simulink library "laser_library"  (Simulink 7.5)
settings: Solver=ode45  StartTime=0.0  StopTime=10.0  RelTol=1e-3
libraries: simulink x3, aerolibutil x3, falter_library x2, aerolibtransform2 x1
settings Model: Creator=elm  LastModifiedBy=falter

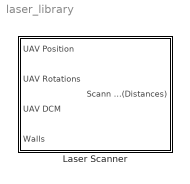
== system laser_library ==
  Laser Scanner : Subsystem  mask{scannerParameters=[0 0 0 1 0 0]}
      mask prompts: scannerParameters "Scanner Parameters"

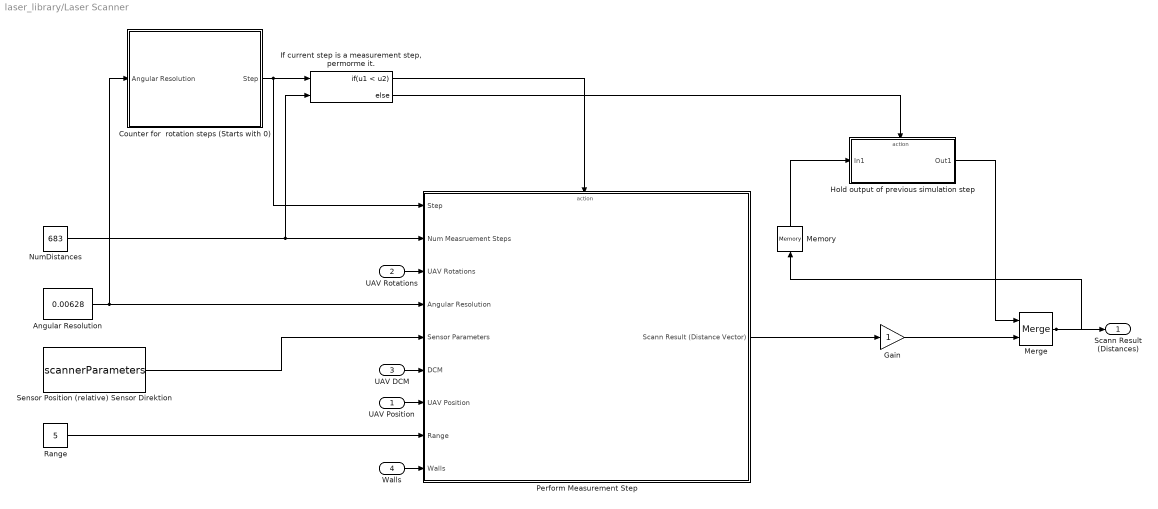
== system laser_library/Laser Scanner ==
  UAV Position : Inport  SampleTime=0.0001
  UAV Rotations : Inport  Port=2  SampleTime=0.0001
  UAV DCM : Inport  Port=3  SampleTime=0.0001
  Walls : Inport  Port=4  SampleTime=0.0001
  Angular Resolution : Constant  Value=0.00628  OutDataType=fixdt(1, 16)  OutScaling=2^0
  Counter for  rotation steps (Starts with 0) : Subsystem
  Gain : Gain  ParameterDataType=fixdt(1, 16)  ParameterScaling=2^0  OutDataType=fixdt(1, 16)  OutScaling=2^0
  Hold output of previous simulation step : Subsystem  TreatAsAtomicUnit=on
  "If current step is a measurement step, permorme it." : If  NumInputs=2  IfExpression=u1 < u2
  Memory : Memory
  Merge : Merge  InitialOutput=0
  NumDistances : Constant  Value=683  OutDataType=fixdt(1, 16)  OutScaling=2^0
  Perform Measurement Step : Subsystem
  Range : Constant  Value=5  OutDataType=fixdt(1, 16)  OutScaling=2^0
  Sensor Position (relative) Sensor Direktion : Constant  Value=scannerParameters  OutDataType=fixdt(1, 16)  OutScaling=2^0
  Scann Result (Distances) : Outport  SampleTime=0.0001
  wires:
  Sensor Position (relative) Sensor Direktion/1 -> Perform Measurement Step/5(Sensor Parameters)
  Walls/1 -> Perform Measurement Step/9(Walls)
  UAV Position/1 -> Perform Measurement Step/7(UAV Position)
  UAV DCM/1 -> Perform Measurement Step/6(DCM)
  UAV Rotations/1 -> Perform Measurement Step/3(UAV Rotations)
  Gain/1 -> Merge/2
  Memory/1 -> Hold output of previous simulation step/1(In1)
  Merge/1 -> Scann Result (Distances)/1, Memory/1
  Hold output of previous simulation step/1(Out1) -> Merge/1
  "If current step is a measurement step, permorme it."/2 -> Hold output of previous simulation step/Action
  Perform Measurement Step/1(Scann Result (Distance Vector)) -> Gain/1
  "If current step is a measurement step, permorme it."/1 -> Perform Measurement Step/Action
  Counter for  rotation steps (Starts with 0)/1(Step) -> Perform Measurement Step/1(Step), "If current step is a measurement step, permorme it."/1
  NumDistances/1 -> Perform Measurement Step/2(Num Measruement Steps), "If current step is a measurement step, permorme it."/2
  Range/1 -> Perform Measurement Step/8(Range)
  Angular Resolution/1 -> Counter for  rotation steps (Starts with 0)/1(Angular Resolution), Perform Measurement Step/4(Angular Resolution)

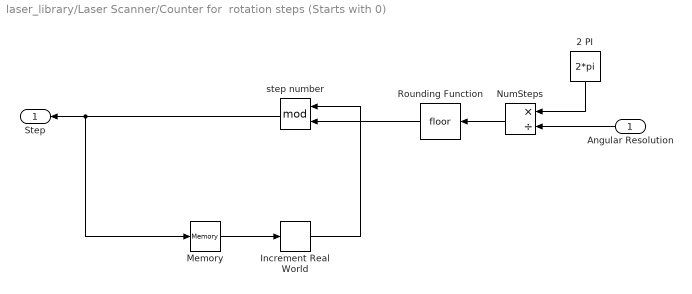
== system laser_library/Laser Scanner/Counter for  rotation steps (Starts with 0) ==
  Angular Resolution : Inport  OutDataType=fixdt(1, 16)  OutScaling=2^0
  2 PI : Constant  Value=2*pi  OutDataType=fixdt(1, 16)  OutScaling=2^0
  Increment Real World : simulink/Additional Math & Discrete/Additional Math: Increment - Decrement/Increment Real World  SystemSampleTime=-1
  Memory : Memory  InheritSampleTime=on
  NumSteps : Product  Inputs=*/  OutDataType=fixdt(1, 16)  OutScaling=2^-10
  Rounding Function : Rounding
  step number : Math  Operator=mod  OutDataType=fixdt(1, 16)  OutScaling=2^0  SaturateOnIntegerOverflow=on
  Step : Outport
  wires:
  Rounding Function/1 -> step number/2
  NumSteps/1 -> Rounding Function/1
  2 PI/1 -> NumSteps/1
  Angular Resolution/1 -> NumSteps/2
  step number/1 -> Memory/1, Step/1
  Increment Real World/1 -> step number/1
  Memory/1 -> Increment Real World/1

== system laser_library/Laser Scanner/Hold output of previous simulation step ==
  In1 : Inport  OutDataType=fixdt(1, 16)  OutScaling=2^0
  Action Port : ActionPort
  Out1 : Outport  OutDataType=fixdt(1, 16)  OutScaling=2^0  InitialOutput=0
  wires:
  In1/1 -> Out1/1

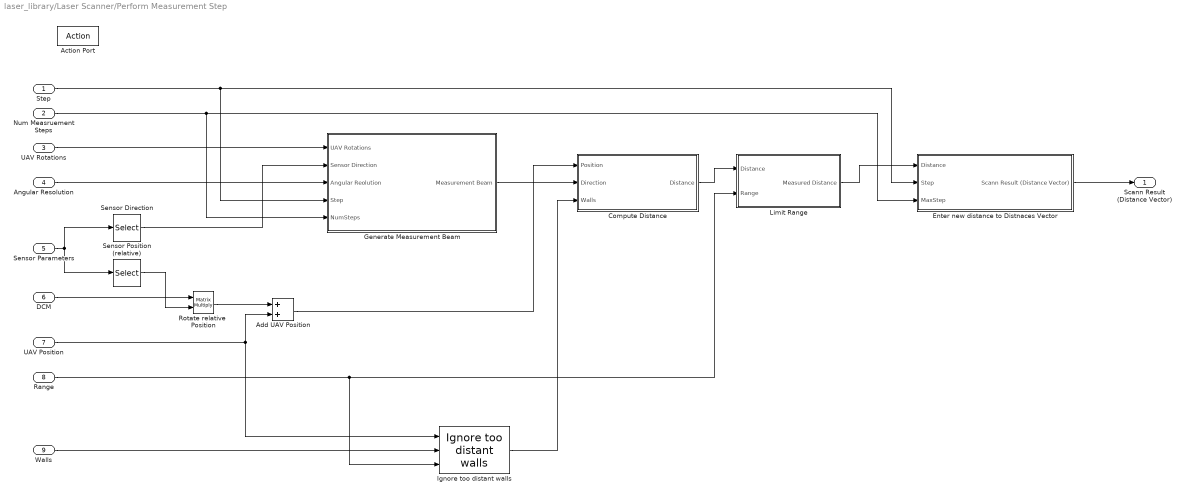
== system laser_library/Laser Scanner/Perform Measurement Step ==
  Step : Inport
  Num Measruement Steps : Inport  Port=2
  UAV Rotations : Inport  Port=3
  Angular Resolution : Inport  Port=4
  Sensor Parameters : Inport  Port=5
  DCM : Inport  Port=6
  UAV Position : Inport  Port=7
  Range : Inport  Port=8
  Walls : Inport  Port=9
  Action Port : ActionPort
  Add UAV Position : Sum  OutDataType=fixdt(1, 16)  OutScaling=2^-10
  Compute Distance : Subsystem
  Enter new distance to Distnaces Vector : Subsystem
  Generate Measurement Beam : Subsystem
  Ignore too distant walls : falter_library/Ignore too distant walls  SystemSampleTime=-1
  Limit Range : Subsystem
  Rotate relative  Position : Product  Multiplication=Matrix(*)  OutDataType=fixdt(1, 16)  OutScaling=2^0  RndMeth=Zero
  Sensor Direction : Selector  InputPortWidth=6  IndexOptions=Index vector (dialog)  Indices=[4 5 6]  OutputSizes=1
  Sensor Position (relative) : Selector  InputPortWidth=6  IndexOptions=Index vector (dialog)  Indices=[1 2 3]  OutputSizes=1
  Scann Result (Distance Vector) : Outport  InitialOutput=0
  wires:
  Walls/1 -> Ignore too distant walls/2
  Ignore too distant walls/1 -> Compute Distance/3(Walls)
  Angular Resolution/1 -> Generate Measurement Beam/3(Angular Reolution)
  Enter new distance to Distnaces Vector/1(Scann Result (Distance Vector)) -> Scann Result (Distance Vector)/1
  UAV Rotations/1 -> Generate Measurement Beam/1(UAV Rotations)
  Num Measruement Steps/1 -> Generate Measurement Beam/5(NumSteps), Enter new distance to Distnaces Vector/3(MaxStep)
  Limit Range/1(Measured Distance) -> Enter new distance to Distnaces Vector/1(Distance)
  Compute Distance/1(Distance) -> Limit Range/1(Distance)
  Range/1 -> Limit Range/2(Range), Ignore too distant walls/3
  Step/1 -> Enter new distance to Distnaces Vector/2(Step), Generate Measurement Beam/4(Step)
  Generate Measurement Beam/1(Measurement Beam) -> Compute Distance/2(Direction)
  Add UAV Position/1 -> Compute Distance/1(Position)
  UAV Position/1 -> Add UAV Position/2, Ignore too distant walls/1
  Sensor Direction/1 -> Generate Measurement Beam/2(Sensor Direction)
  Sensor Parameters/1 -> Sensor Direction/1, Sensor Position (relative)/1
  DCM/1 -> Rotate relative  Position/1
  Sensor Position (relative)/1 -> Rotate relative  Position/2
  Rotate relative  Position/1 -> Add UAV Position/1

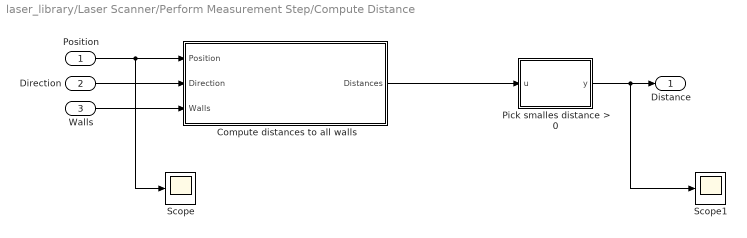
== system laser_library/Laser Scanner/Perform Measurement Step/Compute Distance ==
  Position : Inport  OutDataType=fixdt(1, 16)  OutScaling=2^0
  Direction : Inport  Port=2  OutDataType=fixdt(1, 16)  OutScaling=2^0
  Walls : Inport  Port=3  OutDataType=fixdt(1, 16)  OutScaling=2^0
  Compute distances to all walls : Subsystem  TreatAsAtomicUnit=on
  Pick smalles distance > 0 : Stateflow chart  TreatAsAtomicUnit=on
  Scope : Scope
      settings: YMin=0  YMax=1  SaveName=ScopeData4
  Scope1 : Scope
      settings: YMin=0  YMax=130  SaveName=ScopeData3
  Distance : Outport  OutDataType=fixdt(1, 16)  OutScaling=2^0
  wires:
  Pick smalles distance > 0/1(y) -> Distance/1, Scope1/1
  Compute distances to all walls/1(Distances) -> Pick smalles distance > 0/1(u)
  Position/1 -> Scope/1, Compute distances to all walls/1(Position)
  Direction/1 -> Compute distances to all walls/2(Direction)
  Walls/1 -> Compute distances to all walls/3(Walls)

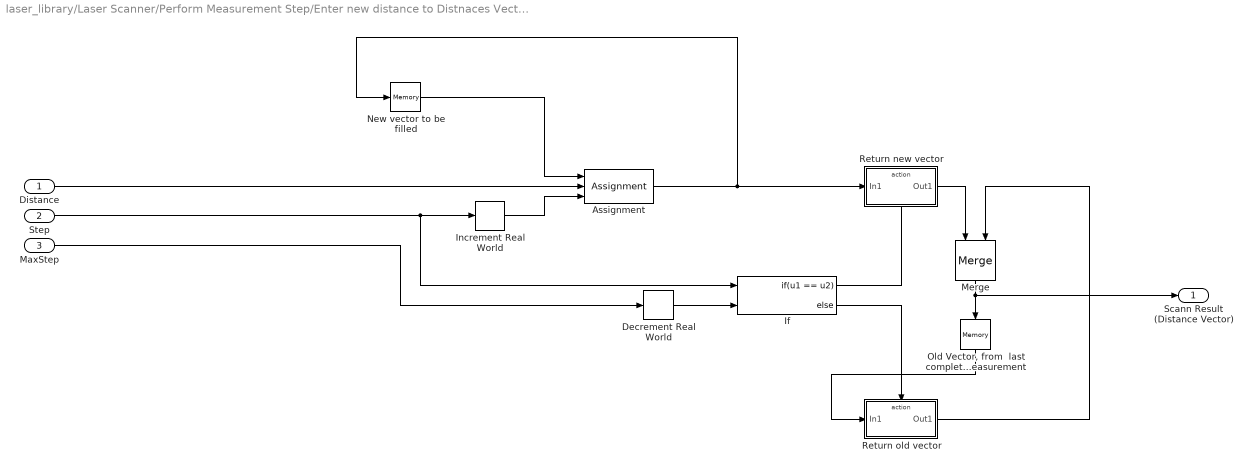
== system laser_library/Laser Scanner/Perform Measurement Step/Enter new distance to Distnaces Vector ==
  Distance : Inport  OutDataType=fixdt(1, 16)  OutScaling=2^0
  Step : Inport  Port=2  OutDataType=fixdt(1, 16)  OutScaling=2^0
  MaxStep : Inport  Port=3  OutDataType=fixdt(1, 16)  OutScaling=2^0
  Assignment : Assignment  IndexOptions=Index vector (port)  Indices=1  OutputSizes=1
  Decrement Real World : simulink/Additional Math & Discrete/Additional Math: Increment - Decrement/Decrement Real World  SystemSampleTime=-1
  If : If  NumInputs=2  IfExpression=u1 == u2
  Increment Real World : simulink/Additional Math & Discrete/Additional Math: Increment - Decrement/Increment Real World  SystemSampleTime=-1
  Merge : Merge  InitialOutput=0
  New vector to be filled : Memory  X0=[0 0 0 0 0 0 0 0 0 0 0 0 0 0 0 0 0 0 0 0 0 0 0 0 0 0 0 0 0 0 0 0 0 0 0 0 0 0 0 0 0 0 0 0 0 0 0 0 0 0 0 0 0 0 0 0 0 0 0 0 0 0 0 0 0 0 0 0 0 0 0 0 0 0 0 0 0 0 0 0 0 0 0 0 0 0 0 0 0 0 0 0 0 0 0 0 0 0 0 0 0 0 0 0 0 0 0 0 0 0 0 0 0 0 0 0 0 0 0 0 0 0 0 0 0 0 0 0 0 0 0 0 0 0 0 0 0 0 0 0 0 0 0 0 0 0 0 0 0 0 0 0 0 0 0 0 0 0 0 0 0 0 0 0 0 0 0 0 0 0 0 0 0 0 0 0 0 0 0 0 0 0 0 0 0 0 0 0 0 0 0 0 0 0 0 0 0 0 0 0 0 0 0 0 0 0 0 0 0 0 0 0 0 0 0 0 0 0 0 0 0 0 0 0 0 0 0 0 0 0 0 0 0 0 0 0 0 0 0 0 0 0 0 0 0 0 0 0 0 0 0 0 0 0 0 0 0 0 0 0 0 0 0 0 0 0 0 0 0 0 0 0 0 0 0 0 0 0 0 0 0 0 0 0 0 0 0 0 0 0 0 0 0 0 0 0 0 0 0 0 0 0 0 0 0 0 0 0 0 0 0 0 0 0 0 0 0 0 0 0 0 0 0 0 0 0 0 0 0 0 0 0 0 0 0 0 0 0 0 0 0 0 0 0 0 0 0 0 0 0 0 0 0 0 0 0 0 0 0 0 0 0 0 0 0 0 0 0 0 0 0 0 0 0 0 0 0 0 0 0 0 0 0 0 0 0 0 0 0 0 0 0 0 0 0 0 0 0 0 0 0 0 0 0 0 0 0 0 0 0 0 0 0 0 0 0 0 0 0 0 0 0 0 0 0 0 0 0 0 0 0 0 0 0 0 0 0 0 0 0 0 0 0 0 0 0 0 0 0 0 0 0 0 0 0 0 0 0 0 0 0 0 0 0 0 0 0 0 0 0 0 0 0 0 0 0 0 0 0 0 0 0 0 0 0 0 0 0 0 0 0 0 0 0 0 0 0 0 0 0 0 0 0 0 0 0 0 0 0 0 0 0 0 0 0 0 0 0 0 0 0 0 0 0 0 0 0 0 0 0 0 0 0 0 0 0 0 0 0 0 0 0 0 0 0 0 0 0 0 0 0 0 0 0 0 0 0 0 0 0 0 0 0 0 0 0 0 0 0 0 0 0 0 0 0 0 0 0 0 0 0 0 0 0 0 0 0 0 0 0 0 0 0 0 0 0 0 0 0 0 0 0 0 0 0 0 0 0 0 0 0 0 0 0 0 0 0 0 0 0 0 0 0 0 0 0 0 0 0 0 0 0 0 0 0 0 0 0 0 0 0 0 0 0 0 0 0 0 0 0 0 0 0 0 0 0 0 0 0 0 0 0 0 0 0 0 0 0 0 0 0 0 0 0 0 0 0 0 0 0 0 0 0]  InheritSampleTime=on
  "Old Vector, from  last complete  measurement" : Memory  X0=[0 0 0 0 0 0 0 0 0 0 0 0 0 0 0 0 0 0 0 0 0 0 0 0 0 0 0 0 0 0 0 0 0 0 0 0 0 0 0 0 0 0 0 0 0 0 0 0 0 0 0 0 0 0 0 0 0 0 0 0 0 0 0 0 0 0 0 0 0 0 0 0 0 0 0 0 0 0 0 0 0 0 0 0 0 0 0 0 0 0 0 0 0 0 0 0 0 0 0 0 0 0 0 0 0 0 0 0 0 0 0 0 0 0 0 0 0 0 0 0 0 0 0 0 0 0 0 0 0 0 0 0 0 0 0 0 0 0 0 0 0 0 0 0 0 0 0 0 0 0 0 0 0 0 0 0 0 0 0 0 0 0 0 0 0 0 0 0 0 0 0 0 0 0 0 0 0 0 0 0 0 0 0 0 0 0 0 0 0 0 0 0 0 0 0 0 0 0 0 0 0 0 0 0 0 0 0 0 0 0 0 0 0 0 0 0 0 0 0 0 0 0 0 0 0 0 0 0 0 0 0 0 0 0 0 0 0 0 0 0 0 0 0 0 0 0 0 0 0 0 0 0 0 0 0 0 0 0 0 0 0 0 0 0 0 0 0 0 0 0 0 0 0 0 0 0 0 0 0 0 0 0 0 0 0 0 0 0 0 0 0 0 0 0 0 0 0 0 0 0 0 0 0 0 0 0 0 0 0 0 0 0 0 0 0 0 0 0 0 0 0 0 0 0 0 0 0 0 0 0 0 0 0 0 0 0 0 0 0 0 0 0 0 0 0 0 0 0 0 0 0 0 0 0 0 0 0 0 0 0 0 0 0 0 0 0 0 0 0 0 0 0 0 0 0 0 0 0 0 0 0 0 0 0 0 0 0 0 0 0 0 0 0 0 0 0 0 0 0 0 0 0 0 0 0 0 0 0 0 0 0 0 0 0 0 0 0 0 0 0 0 0 0 0 0 0 0 0 0 0 0 0 0 0 0 0 0 0 0 0 0 0 0 0 0 0 0 0 0 0 0 0 0 0 0 0 0 0 0 0 0 0 0 0 0 0 0 0 0 0 0 0 0 0 0 0 0 0 0 0 0 0 0 0 0 0 0 0 0 0 0 0 0 0 0 0 0 0 0 0 0 0 0 0 0 0 0 0 0 0 0 0 0 0 0 0 0 0 0 0 0 0 0 0 0 0 0 0 0 0 0 0 0 0 0 0 0 0 0 0 0 0 0 0 0 0 0 0 0 0 0 0 0 0 0 0 0 0 0 0 0 0 0 0 0 0 0 0 0 0 0 0 0 0 0 0 0 0 0 0 0 0 0 0 0 0 0 0 0 0 0 0 0 0 0 0 0 0 0 0 0 0 0 0 0 0 0 0 0 0 0 0 0 0 0 0 0 0 0 0 0 0 0 0 0 0 0 0 0 0 0 0 0 0 0 0 0 0 0 0 0 0 0 0 0 0 0 0 0 0 0 0 0 0 0 0 0 0 0 0 0 0 0 0 0 0 0 0 0 0 0 0 0 0 0 0 0 0 0 0 0 0 0]  InheritSampleTime=on
  Return new vector : Subsystem  TreatAsAtomicUnit=on
  Return old vector : Subsystem  TreatAsAtomicUnit=on
  Scann Result (Distance Vector) : Outport  OutDataType=fixdt(1, 16)  OutScaling=2^0
  wires:
  Decrement Real World/1 -> If/2
  Return old vector/1(Out1) -> Merge/2
  Merge/1 -> Scann Result (Distance Vector)/1, "Old Vector, from  last complete  measurement"/1
  Return new vector/1(Out1) -> Merge/1
  Distance/1 -> Assignment/2
  "Old Vector, from  last complete  measurement"/1 -> Return old vector/1(In1)
  If/2 -> Return old vector/Action
  If/1 -> Return new vector/Action
  MaxStep/1 -> Decrement Real World/1
  Assignment/1 -> New vector to be filled/1, Return new vector/1(In1)
  Step/1 -> If/1, Increment Real World/1
  New vector to be filled/1 -> Assignment/1
  Increment Real World/1 -> Assignment/3

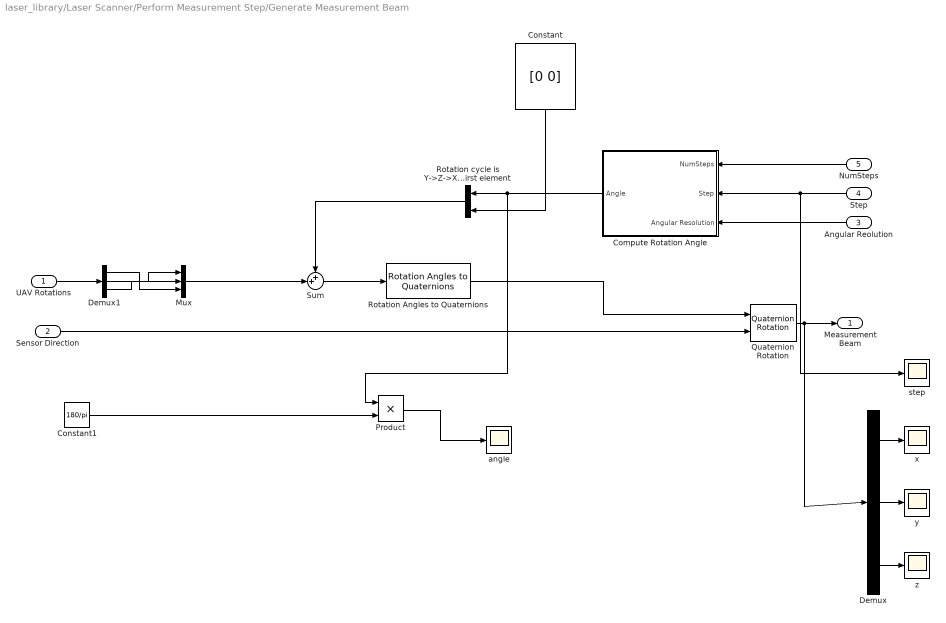
== system laser_library/Laser Scanner/Perform Measurement Step/Generate Measurement Beam ==
  UAV Rotations : Inport
  Sensor Direction : Inport  Port=2
  Angular Reolution : Inport  Port=3
  Step : Inport  Port=4
  NumSteps : Inport  Port=5
  Compute Rotation Angle : Subsystem
  Constant : Constant  Value=[0 0]  OutDataType=fixdt(1, 16)  OutScaling=2^0
  Constant1 : Constant  Value=180/pi  OutDataType=fixdt(1, 16)  OutScaling=2^0
  Demux : Demux  Outputs=3
  Demux1 : Demux  Outputs=3
  Mux : Mux  Inputs=3
  Product : Product  OutDataType=fixdt(1, 16)  OutScaling=2^0  RndMeth=Zero
  Quaternion Rotation : aerolibutil/Quaternion Rotation  SystemSampleTime=-1
  Rotation Angles to Quaternions : aerolibtransform2/Rotation Angles to Quaternions  SystemSampleTime=-1  rotationOrder=YZX
  Rotation cycle is Y->Z->X y (vertical ax. in sim!) is first element : Concatenate  Mode=Vector
  Sum : Sum  Inputs=++|  OutDataType=fixdt(1, 16)  OutScaling=2^0
  angle : Scope
      settings: YMin=0  YMax=700  SaveName=ScopeData5
  step : Scope
      settings: YMin=0  YMax=700
  x : Scope
      settings: YMin=-2.5  YMax=2.5  SaveName=ScopeData2
  y : Scope
      settings: YMin=-1  YMax=1  SaveName=ScopeData4
  z : Scope
      settings: YMin=-1  YMax=1  SaveName=ScopeData3
  Measurement Beam : Outport
  wires:
  NumSteps/1 -> Compute Rotation Angle/1(NumSteps)
  Step/1 -> Compute Rotation Angle/2(Step), step/1
  Angular Reolution/1 -> Compute Rotation Angle/3(Angular Resolution)
  Sensor Direction/1 -> Quaternion Rotation/2
  Sum/1 -> Rotation Angles to Quaternions/1
  Rotation Angles to Quaternions/1 -> Quaternion Rotation/1
  Rotation cycle is Y->Z->X y (vertical ax. in sim!) is first element/1 -> Sum/1
  Demux/1 -> x/1
  Demux/2 -> y/1
  Demux/3 -> z/1
  Quaternion Rotation/1 -> Measurement Beam/1, Demux/1
  Compute Rotation Angle/1(Angle) -> Rotation cycle is Y->Z->X y (vertical ax. in sim!) is first element/1, Product/1
  Constant/1 -> Rotation cycle is Y->Z->X y (vertical ax. in sim!) is first element/2
  Constant1/1 -> Product/2
  Product/1 -> angle/1
  UAV Rotations/1 -> Demux1/1
  Demux1/1 -> Mux/3
  Demux1/2 -> Mux/1
  Demux1/3 -> Mux/2
  Mux/1 -> Sum/2

== system laser_library/Laser Scanner/Perform Measurement Step/Limit Range ==
  Distance : Inport  OutDataType=fixdt(1, 16)  OutScaling=2^0
  Range : Inport  Port=2  OutDataType=fixdt(1, 16)  OutScaling=2^0
  If : If  NumInputs=2  IfExpression=u1 <= u2
  If Action Subsystem : Subsystem  TreatAsAtomicUnit=on
  If Action Subsystem1 : Subsystem  TreatAsAtomicUnit=on
  Merge : Merge  InitialOutput=0
  Measured Distance : Outport  OutDataType=fixdt(1, 16)  OutScaling=2^0
  wires:
  Merge/1 -> Measured Distance/1
  If Action Subsystem1/1(Distance=0) -> Merge/2
  If Action Subsystem/1(Out) -> Merge/1
  If/2 -> If Action Subsystem1/Action
  If/1 -> If Action Subsystem/Action
  Range/1 -> If/2
  Distance/1 -> If Action Subsystem/1(In), If/1

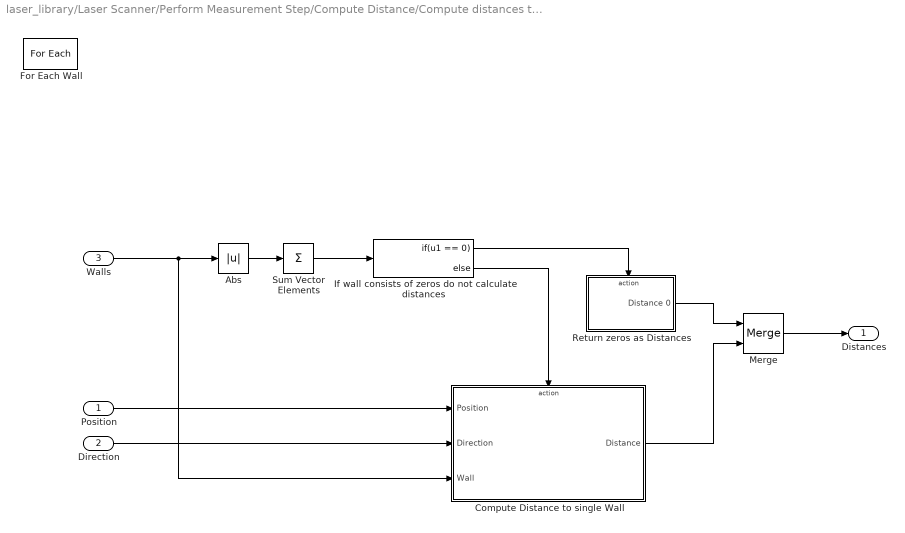
== system laser_library/Laser Scanner/Perform Measurement Step/Compute Distance/Compute distances to all walls ==
  Position : Inport  OutDataType=fixdt(1, 16)  OutScaling=2^0  Partition=off
  Direction : Inport  Port=2  OutDataType=fixdt(1, 16)  OutScaling=2^0  Partition=off
  Walls : Inport  Port=3  OutDataType=fixdt(1, 16)  OutScaling=2^0  Partition=on  PartitionDimension=1  PartitionWidth=1
  Abs : Abs  OutDataType=fixdt(1, 16)  OutScaling=2^0
  Compute Distance to single Wall : Subsystem
  For Each Wall : ForEach  DisableCoverage=on  IndexMode=One-based
  If wall consists of zeros do not calculate distances : If  IfExpression=u1 == 0
  Merge : Merge  InitialOutput=0
  Return zeros as Distances : Subsystem  TreatAsAtomicUnit=on
  Sum Vector Elements : Sum  Inputs=+  OutDataType=fixdt(1, 16)  OutScaling=2^-10
  Distances : Outport  OutDataType=fixdt(1, 16)  OutScaling=2^0  ConcatenationDimension=1
  wires:
  If wall consists of zeros do not calculate distances/2 -> Compute Distance to single Wall/Action
  Compute Distance to single Wall/1(Distance) -> Merge/2
  Sum Vector Elements/1 -> If wall consists of zeros do not calculate distances/1
  Merge/1 -> Distances/1
  Return zeros as Distances/1(Distance 0) -> Merge/1
  Position/1 -> Compute Distance to single Wall/1(Position)
  Direction/1 -> Compute Distance to single Wall/2(Direction)
  Walls/1 -> Compute Distance to single Wall/3(Wall), Abs/1
  If wall consists of zeros do not calculate distances/1 -> Return zeros as Distances/Action
  Abs/1 -> Sum Vector Elements/1

== system laser_library/Laser Scanner/Perform Measurement Step/Enter new distance to Distnaces Vector/Return new vector ==
  In1 : Inport  OutDataType=fixdt(1, 16)  OutScaling=2^0
  Action Port : ActionPort
  Out1 : Outport  OutDataType=fixdt(1, 16)  OutScaling=2^0  InitialOutput=0
  wires:
  In1/1 -> Out1/1

== system laser_library/Laser Scanner/Perform Measurement Step/Enter new distance to Distnaces Vector/Return old vector ==
  In1 : Inport  OutDataType=fixdt(1, 16)  OutScaling=2^0
  Action Port : ActionPort
  Out1 : Outport  OutDataType=fixdt(1, 16)  OutScaling=2^0  InitialOutput=0
  wires:
  In1/1 -> Out1/1

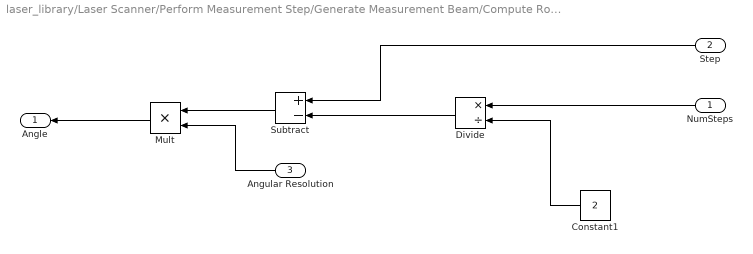
== system laser_library/Laser Scanner/Perform Measurement Step/Generate Measurement Beam/Compute Rotation Angle ==
  NumSteps : Inport
  Step : Inport  Port=2
  Angular Resolution : Inport  Port=3
  Constant1 : Constant  Value=2  OutDataType=fixdt(1, 16)  OutScaling=2^0
  Divide : Product  Inputs=*/  OutDataType=fixdt(1, 16)  OutScaling=2^-10
  Mult : Product  OutDataType=fixdt(1, 16)  OutScaling=2^0  RndMeth=Zero
  Subtract : Sum  Inputs=+-  OutDataType=fixdt(1, 16)  OutScaling=2^-10
  Angle : Outport  OutDataType=fixdt(1, 16)  OutScaling=2^0
  wires:
  Angular Resolution/1 -> Mult/2
  Subtract/1 -> Mult/1
  Divide/1 -> Subtract/2
  Constant1/1 -> Divide/2
  Step/1 -> Subtract/1
  NumSteps/1 -> Divide/1
  Mult/1 -> Angle/1

== system laser_library/Laser Scanner/Perform Measurement Step/Limit Range/If Action Subsystem ==
  In : Inport  OutDataType=fixdt(1, 16)  OutScaling=2^0
  Action Port : ActionPort
  Out : Outport  OutDataType=fixdt(1, 16)  OutScaling=2^0  InitialOutput=0
  wires:
  In/1 -> Out/1

== system laser_library/Laser Scanner/Perform Measurement Step/Limit Range/If Action Subsystem1 ==
  Action Port : ActionPort
  Constant : Constant  Value=0  OutDataType=fixdt(1, 16)  OutScaling=2^0
  Distance=0 : Outport  OutDataType=fixdt(1, 16)  OutScaling=2^0  InitialOutput=0
  wires:
  Constant/1 -> Distance=0/1

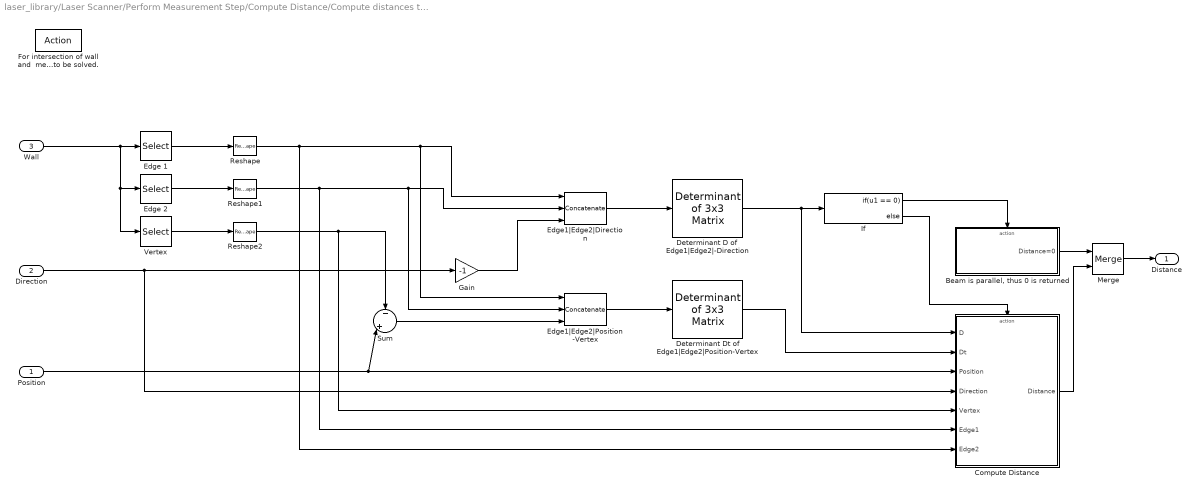
== system laser_library/Laser Scanner/Perform Measurement Step/Compute Distance/Compute distances to all walls/Compute Distance to single Wall ==
  Position : Inport  OutDataType=fixdt(1, 16)  OutScaling=2^0
  Direction : Inport  Port=2  OutDataType=fixdt(1, 16)  OutScaling=2^0
  Wall : Inport  Port=3  OutDataType=fixdt(1, 16)  OutScaling=2^0
  "For intersection of wall and  measurment beam, the sys. of lin. equ. Vertex + r*Edge1 + f*Edge2 = Position + t*Direction needs to be solved." : ActionPort
  "Beam is parallel, thus 0 is returned" : Subsystem  TreatAsAtomicUnit=on
  Compute Distance : Subsystem  TreatAsAtomicUnit=on
  Determinant D of  Edge1|Edge2|-Direction : aerolibutil/Determinant of 3x3 Matrix  SystemSampleTime=-1
  Determinant Dt of Edge1|Edge2|Position-Vertex : aerolibutil/Determinant of 3x3 Matrix  SystemSampleTime=-1
  Edge 1 : Selector  NumberOfDimensions=2  InputPortWidth=3  IndexOptions=Select all,Index vector (dialog)  Indices=[1 2 3],[4 5 6]  OutputSizes=1,1
  Edge 2 : Selector  NumberOfDimensions=2  InputPortWidth=3  IndexOptions=Select all,Index vector (dialog)  Indices=[1 2 3],[7 8 9]  OutputSizes=1,1
  Edge1|Edge2|Direction : Concatenate  NumInputs=3  Mode=Multidimensional array  ConcatenateDimension=2
  Edge1|Edge2|Position-Vertex : Concatenate  NumInputs=3  Mode=Multidimensional array  ConcatenateDimension=2
  Gain : Gain  Gain=-1  ParameterDataType=fixdt(1, 16)  ParameterScaling=2^0  OutDataType=fixdt(1, 16)  OutScaling=2^0
  If : If  IfExpression=u1 == 0
  Merge : Merge  InitialOutput=0
  Reshape : Reshape  OutputDimensionality=Column vector (2-D)
  Reshape1 : Reshape  OutputDimensionality=Column vector (2-D)
  Reshape2 : Reshape  OutputDimensionality=Column vector (2-D)
  Sum : Sum  Inputs=-||+|  OutDataType=fixdt(1, 16)  OutScaling=2^0
  Vertex : Selector  NumberOfDimensions=2  InputPortWidth=3  IndexOptions=Select all,Index vector (dialog)  Indices=[1 2 3],[1 2 3]  OutputSizes=1,1
  Distance : Outport  OutDataType=fixdt(1, 16)  OutScaling=2^0  InitialOutput=0
  wires:
  If/2 -> Compute Distance/Action
  If/1 -> "Beam is parallel, thus 0 is returned"/Action
  Merge/1 -> Distance/1
  Compute Distance/1(Distance) -> Merge/2
  "Beam is parallel, thus 0 is returned"/1(Distance=0) -> Merge/1
  Determinant Dt of Edge1|Edge2|Position-Vertex/1 -> Compute Distance/2(Dt)
  Determinant D of  Edge1|Edge2|-Direction/1 -> If/1, Compute Distance/1(D)
  Reshape2/1 -> Compute Distance/5(Vertex), Sum/1
  Vertex/1 -> Reshape2/1
  Edge1|Edge2|Position-Vertex/1 -> Determinant Dt of Edge1|Edge2|Position-Vertex/1
  Sum/1 -> Edge1|Edge2|Position-Vertex/3
  Position/1 -> Compute Distance/3(Position), Sum/2
  Gain/1 -> Edge1|Edge2|Direction/3
  Direction/1 -> Compute Distance/4(Direction), Gain/1
  Reshape1/1 -> Compute Distance/6(Edge1), Edge1|Edge2|Position-Vertex/2, Edge1|Edge2|Direction/2
  Reshape/1 -> Compute Distance/7(Edge2), Edge1|Edge2|Position-Vertex/1, Edge1|Edge2|Direction/1
  Edge 2/1 -> Reshape1/1
  Edge 1/1 -> Reshape/1
  Edge1|Edge2|Direction/1 -> Determinant D of  Edge1|Edge2|-Direction/1
  Wall/1 -> Vertex/1, Edge 2/1, Edge 1/1

== system laser_library/Laser Scanner/Perform Measurement Step/Compute Distance/Compute distances to all walls/Return zeros as Distances ==
  Action Port : ActionPort
  Constant : Constant  Value=0  OutDataType=fixdt(1, 16)  OutScaling=2^0
  Distance 0 : Outport  OutDataType=fixdt(1, 16)  OutScaling=2^0  InitialOutput=0
  wires:
  Constant/1 -> Distance 0/1

== system laser_library/Laser Scanner/Perform Measurement Step/Compute Distance/Compute distances to all walls/Compute Distance to single Wall/Beam is parallel, thus 0 is returned ==
  Action Port : ActionPort
  Constant : Constant  Value=0  OutDataType=fixdt(1, 16)  OutScaling=2^0
  Distance=0 : Outport  OutDataType=fixdt(1, 16)  OutScaling=2^0  InitialOutput=0
  wires:
  Constant/1 -> Distance=0/1

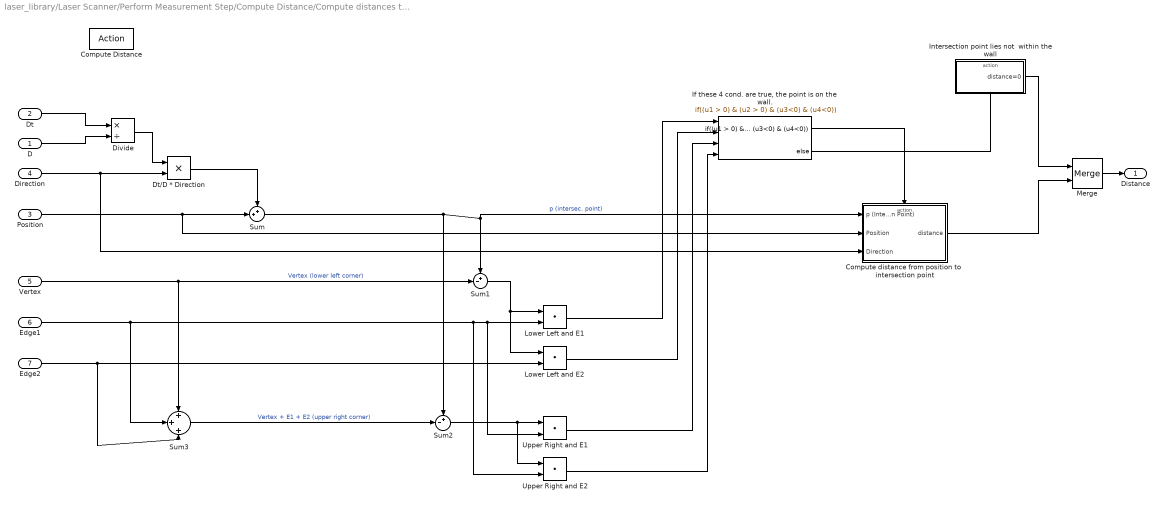
== system laser_library/Laser Scanner/Perform Measurement Step/Compute Distance/Compute distances to all walls/Compute Distance to single Wall/Compute Distance ==
  D : Inport  OutDataType=fixdt(1, 16)  OutScaling=2^0
  Dt : Inport  Port=2  OutDataType=fixdt(1, 16)  OutScaling=2^0
  Position : Inport  Port=3  OutDataType=fixdt(1, 16)  OutScaling=2^0
  Direction : Inport  Port=4  OutDataType=fixdt(1, 16)  OutScaling=2^0
  Vertex : Inport  Port=5  OutDataType=fixdt(1, 16)  OutScaling=2^0
  Edge1 : Inport  Port=6  OutDataType=fixdt(1, 16)  OutScaling=2^0
  Edge2 : Inport  Port=7  OutDataType=fixdt(1, 16)  OutScaling=2^0
  Compute Distance : ActionPort
  Compute distance from position to  intersection point : Subsystem  TreatAsAtomicUnit=on
  Divide : Product  Inputs=*/  OutDataType=fixdt(1, 16)  OutScaling=2^-10
  Dt/D * Direction : Product  OutDataType=fixdt(1, 16)  OutScaling=2^0  RndMeth=Zero
  "If these 4 cond. are true, the point is on the wall." : If  NumInputs=4  IfExpression=(u1 > 0) & (u2 > 0) & (u3<0) & (u4<0)
  Intersection point lies not  within the wall : Subsystem  TreatAsAtomicUnit=on
  Lower Left and E1 : DotProduct  OutDataType=fixdt(1, 16)  OutScaling=2^-10  InputSameDT=on  OutDataTypeStr=Inherit: Inherit via internal rule
  Lower Left and E2 : DotProduct  OutDataType=fixdt(1, 16)  OutScaling=2^-10  InputSameDT=on  OutDataTypeStr=Inherit: Inherit via internal rule
  Merge : Merge  InitialOutput=0
  Sum : Sum  Inputs=++|  OutDataType=fixdt(1, 16)  OutScaling=2^0
  Sum1 : Sum  Inputs=+-|  OutDataType=fixdt(1, 16)  OutScaling=2^0
  Sum2 : Sum  Inputs=+-|  OutDataType=fixdt(1, 16)  OutScaling=2^0
  Sum3 : Sum  Inputs=+|+|+  OutDataType=fixdt(1, 16)  OutScaling=2^0
  Upper Right and E1 : DotProduct  OutDataType=fixdt(1, 16)  OutScaling=2^-10  InputSameDT=on  OutDataTypeStr=Inherit: Inherit via internal rule
  Upper Right and E2 : DotProduct  OutDataType=fixdt(1, 16)  OutScaling=2^-10  InputSameDT=on  OutDataTypeStr=Inherit: Inherit via internal rule
  Distance : Outport  OutDataType=fixdt(1, 16)  OutScaling=2^0  InitialOutput=0
  wires:
  Compute distance from position to  intersection point/1(distance) -> Merge/2
  Intersection point lies not  within the wall/1(distance=0) -> Merge/1
  Merge/1 -> Distance/1
  "If these 4 cond. are true, the point is on the wall."/2 -> Intersection point lies not  within the wall/Action
  "If these 4 cond. are true, the point is on the wall."/1 -> Compute distance from position to  intersection point/Action
  Upper Right and E2/1 -> "If these 4 cond. are true, the point is on the wall."/4
  Upper Right and E1/1 -> "If these 4 cond. are true, the point is on the wall."/3
  Sum2/1 -> Upper Right and E2/1, Upper Right and E1/1
  Sum3/1 -> Sum2/2  "Vertex + E1 + E2 (upper right corner)"
  Lower Left and E2/1 -> "If these 4 cond. are true, the point is on the wall."/2
  Lower Left and E1/1 -> "If these 4 cond. are true, the point is on the wall."/1
  Edge2/1 -> Sum3/3, Lower Left and E2/2
  Edge1/1 -> Upper Right and E2/2, Upper Right and E1/2, Lower Left and E1/2, Sum3/2
  Sum1/1 -> Lower Left and E1/1, Lower Left and E2/1
  Vertex/1 -> Sum3/1, Sum1/2  "Vertex (lower left corner)"
  Dt/D * Direction/1 -> Sum/1
  Direction/1 -> Compute distance from position to  intersection point/3(Direction), Dt/D * Direction/2
  Divide/1 -> Dt/D * Direction/1
  Position/1 -> Compute distance from position to  intersection point/2(Position), Sum/2
  Dt/1 -> Divide/1
  D/1 -> Divide/2
  Sum/1 -> Compute distance from position to  intersection point/1(p (Intersection Point)), Sum1/1, Sum2/1  "p (intersec. point)"

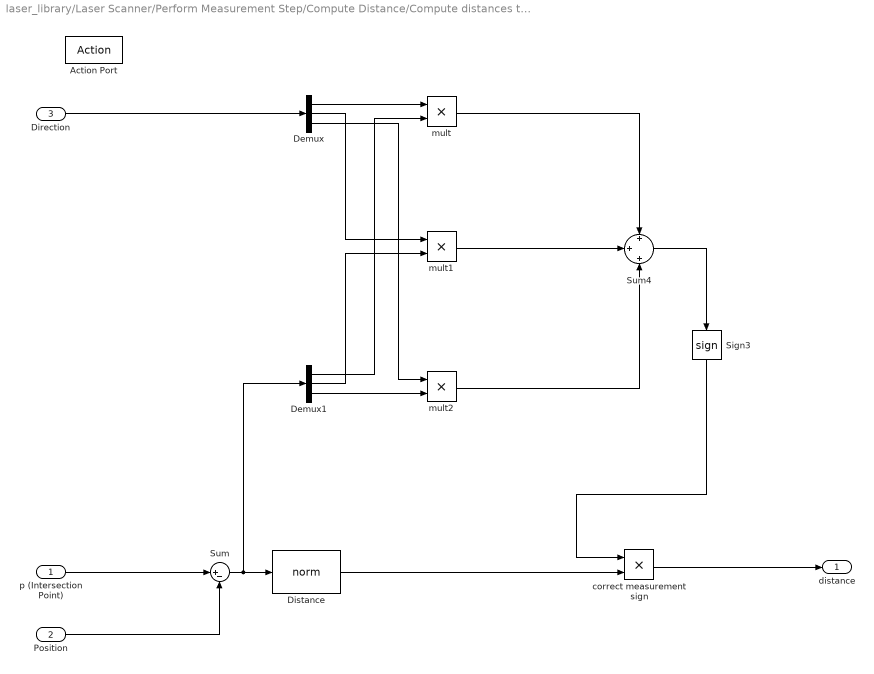
== system laser_library/Laser Scanner/Perform Measurement Step/Compute Distance/Compute distances to all walls/Compute Distance to single Wall/Compute Distance/Compute distance from position to  intersection point ==
  p (Intersection Point) : Inport  OutDataType=fixdt(1, 16)  OutScaling=2^0
  Position : Inport  Port=2  OutDataType=fixdt(1, 16)  OutScaling=2^0
  Direction : Inport  Port=3  OutDataType=fixdt(1, 16)  OutScaling=2^0
  Action Port : ActionPort
  Demux : Demux  Outputs=3
  Demux1 : Demux  Outputs=3
  Distance : falter_library/norm  SystemSampleTime=-1
  Sign3 : Signum
  Sum : Sum  Inputs=|+-  OutDataType=fixdt(1, 16)  OutScaling=2^0
  Sum4 : Sum  Inputs=+|+|+  OutDataType=fixdt(1, 16)  OutScaling=2^0
  correct measurement sign : Product  OutDataType=fixdt(1, 16)  OutScaling=2^0  RndMeth=Zero
  mult : Product  OutDataType=fixdt(1, 16)  OutScaling=2^0  RndMeth=Zero
  mult1 : Product  OutDataType=fixdt(1, 16)  OutScaling=2^0  RndMeth=Zero
  mult2 : Product  OutDataType=fixdt(1, 16)  OutScaling=2^0  RndMeth=Zero
  distance : Outport  OutDataType=fixdt(1, 16)  OutScaling=2^0  InitialOutput=0
  wires:
  Demux1/3 -> mult2/2
  Demux1/2 -> mult1/2
  Demux1/1 -> mult/2
  Demux/3 -> mult2/1
  Demux/2 -> mult1/1
  Demux/1 -> mult/1
  Sign3/1 -> correct measurement sign/1
  Sum4/1 -> Sign3/1
  mult2/1 -> Sum4/3
  mult1/1 -> Sum4/2
  correct measurement sign/1 -> distance/1
  Distance/1 -> correct measurement sign/2
  mult/1 -> Sum4/1
  Direction/1 -> Demux/1
  Sum/1 -> Demux1/1, Distance/1
  Position/1 -> Sum/2
  p (Intersection Point)/1 -> Sum/1

== system laser_library/Laser Scanner/Perform Measurement Step/Compute Distance/Compute distances to all walls/Compute Distance to single Wall/Compute Distance/Intersection point lies not  within the wall ==
  Action Port : ActionPort
  Constant : Constant  Value=0  OutDataType=fixdt(1, 16)  OutScaling=2^0
  distance=0 : Outport  OutDataType=fixdt(1, 16)  OutScaling=2^0  InitialOutput=0
  wires:
  Constant/1 -> distance=0/1

== matlab function Laser Scanner/Perform Measurement Step/Compute Distance/Pick smalles distance > 0 ==
  data: u input double; y output double
function y = fcn(u)
%#eml

[len wid] = size(u);

inf = 9999999;

min = inf;

for i=1:len,
    if ((u(i) > 0) & (min > u(i)))
        min = u(i);
    end
end

if (min == inf)
    y = 0;
else
    y = min;
end
